simulink model "Final_Simulink_Model_assignment_2"  (R2022b)
settings: Solver=FixedStepAuto  StartTime=0.0  StopTime=inf  FixedStep=1e-3  RelTol=1e-3  EnableMultiTasking=on
undefined symbols (not defined in the file): ATR_PULSE_WIDTH, ATR_PUSLE_WIDTH, D0, D1, D10, D11, D12, D13, D2, D3, D4, D5, D6, D7, D8, D9, LRL, magnitude, PTA0, PTA1, PTA2, PTB23, PTB9, PTC16, PTC17, PTC2, PTC3, PTC4, PTD0, PTD1, PTD2, PTD3, REF_PERIOD, REF_PREIOD, VENT_PULSE_WIDTH
libraries: frdmk64flib x19, etargetslib x9, dspstat3 x1
settings Model: ExtModeTrigDuration=5  Creator=clara  LastModifiedBy=dinghao
settings OptimizationCC: EnhancedBackFolding=on  PassReuseOutputArgsAs=Individual arguments  ZeroExternalMemoryAtStartup=off  ZeroInternalMemoryAtStartup=off  MaxStackSize=64  OptimizeBlockOrder=speed  DifferentSizesBufferReuse=on  OptimizationCustomize=off  EfficientTunableParamExpr=on
settings DebuggingCC: ParameterTunabilityLossMsg=error
settings HardwareCC: ProdBitPerPointer=32  ProdBitPerSizeT=32  ProdBitPerPtrDiffT=32  ProdLargestAtomicInteger=Long  ProdLargestAtomicFloat=Double  ProdWordSize=32  ProdHWDeviceType=ARM Compatible->ARM Cortex
settings ModelReferenceCC: EnableRefExpFcnMdlSchedulingChecks=on
settings SFSimCC: MATLABDynamicMemAlloc=off
settings RTWCC: Description=Embedded Coder  SystemTargetFile=ert.tlc  HardwareBoard=NXP FRDM-K64F  TLCOptions="-aInlineSetEventsForThisBaseRateFcn=TLC_FALSE -aSuppressMultiTaskScheduler=TLC_FALSE  -aRateBasedStepFcn=0"  TemplateMakefile=ert_default_tmf  Toolchain=GNU Tools for ARM Embedded Processors
settings CodeAppCC: ForceParamTrailComments=on  IgnoreCustomStorageClasses=off  OperatorAnnotations=on  SimulinkDataObjDesc=on  SFDataObjDesc=on  InsertBlockDesc=on
settings ERTTargetCC: ExtModeTransport=4  ExtModeMexFile=sendToCommService

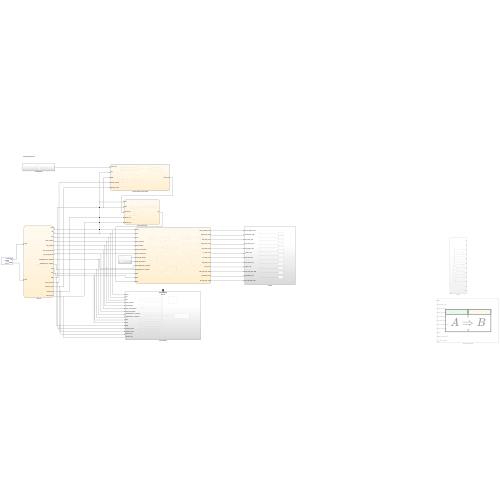
[thumbnail: Simulink's stored preview of the top-level diagram]
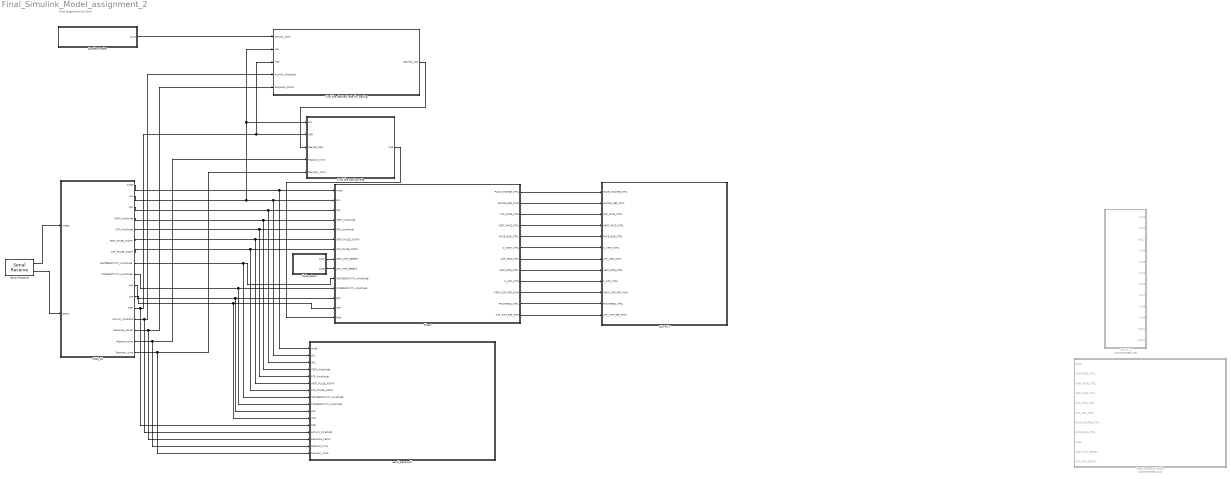
== system Final_Simulink_Model_assignment_2 ==
  note: Find target activity level
  Accelerometer : Subsystem
  COM_IN : Stateflow chart  TreatAsAtomicUnit=on
  Chart : Stateflow chart  TreatAsAtomicUnit=on
      settings: PortSchema="{\"entries\":[{\"content\":{\"sides\":[{\"content\":{\"connectorIds\":[\"In10\",\"In1\",\"In6\",\"In2\",\"In3\",\"In4\",\"In5\",\"In7\",\"In8\",\"In9\",\"In11\",\"In12\",\"In13\",\"In14\"]},\"type\":\"ConnectorPlacement.EquallySpacedRectSide\",\"uuid\":\"411cfc43-89c3-4653-9fab-0da98be593d3\"},{\"content\":{\"connectorIds\":[\"Out1\",\"Out2\",\"Out3\",\"Out4\",\"Out5\",\"Out6\",\"Out7\",\"Out8\",\"Out9\",\"Out10\",\"Out11\",\"Out12\"],\"side\":\"RIGHT\"},\"type\":\"ConnectorPlacement.EquallySpacedRectSide\",\"uuid\":\"ad1683f7-26aa-4767-b656-f3b731cb8235\"},{\"content\":{\"connectorIds\":[],\"side\":\"TOP\"},\"type\":\"ConnectorPlacement.EquallySpacedRectSide\",\"uuid\":\"fbccba07-c1cc-4c9f-8e56-0bdfb6912bb8\"}]},\"type\":\"ConnectorPlacement.EquallySpacedConnector\",\"uuid\":\"0c618a7f-9484-4de3-a6ac-3c8308721375\"}],\"packageUris\":[\"http://schema.mathworks.com/mf0/Connector/R2020b\"],\"version\":\"1.0\"}"
  Find the desired rate for pacing : Stateflow chart  TreatAsAtomicUnit=on
  Find the pacing rate : Stateflow chart  TreatAsAtomicUnit=on
  INPUT 1 : Subsystem  Commented=on
  OUTPUT : Subsystem
  Requirements Table : Requirements Table  Commented=on  TreatAsAtomicUnit=on
  Serial Receive : frdmk64flib/Serial Receive  SCIModule=0  Baudrate=uint32(9600)  Parity=None  StopBits=1  HardwareFlowControl=None  ByteOrder=LittleEndian  DataType=uint8  DataLength=49  BlockingMode=off  OutputStatus=on  SampleTime=-1
  Subsystem : Subsystem
  send_params() : Subsystem
  wires:
  Chart/7(ATR_GND_CTRL) -> OUTPUT/7(ATR_GND_CTRL)
  Chart/3(ATR_PACE_CTRL) -> OUTPUT/3(ATR_PACE_CTRL)
  Chart/6(Z_VENT_CTRL) -> OUTPUT/6(Z_VENT_CTRL)
  Chart/8(VENT_GND_CTRL) -> OUTPUT/8(VENT_GND_CTRL)
  Chart/5(PACE_GND_CTRL) -> OUTPUT/5(PACE_GND_CTRL)
  Chart/9(Z_ATR_CTRL) -> OUTPUT/9(Z_ATR_CTRL)
  Chart/2(PACING_REF_PWM) -> OUTPUT/2(PACING_REF_PWM)
  Chart/1(PACE_CHARGE_CTRL) -> OUTPUT/1(PACE_CHARGE_CTRL)
  Chart/4(VENT_PACE_CTRL) -> OUTPUT/4(VENT_PACE_CTRL)
  Chart/11(FRONTEND_CTRL) -> OUTPUT/11(FRONTEND_CTRL)
  Chart/10(VENT_CMP_REF_PWM) -> OUTPUT/10(VENT_CMP_REF_PWM)
  Chart/12(ATR_CMP_REF_PWM) -> OUTPUT/12(ATR_CMP_REF_PWM)
  Serial Receive/1 -> COM_IN/1(rxdata)
  Serial Receive/2 -> COM_IN/2(status)
  Accelerometer/1(Out1) -> Find the desired rate for pacing/1(Activity_level)
  COM_IN/2(LRL) -> send_params()/2(LRL), Chart/1(LRL), Find the pacing rate/1(LRL), Find the desired rate for pacing/2(LRL)
  COM_IN/12(MSR) -> send_params()/12(MSR), Find the pacing rate/2(MSR), Find the desired rate for pacing/3(MSR)
  COM_IN/13(Activity_threshold) -> send_params()/13(Activity_threshold), Find the desired rate for pacing/4(Activity_threshold)
  COM_IN/14(Response_Factor) -> send_params()/14(Response_Factor), Find the desired rate for pacing/5(Response_Factor)
  Find the desired rate for pacing/1(Desired_rate) -> Find the pacing rate/3(Desired_rate)
  COM_IN/15(Reaction_time) -> send_params()/15(Reaction_time), Find the pacing rate/4(Reaction_time)
  COM_IN/16(Recovery_time) -> send_params()/16(Recovery_time), Find the pacing rate/5(Recovery_time)
  Find the pacing rate/1(rate) -> Chart/14(Rate)
  COM_IN/1(mode) -> send_params()/1(mode), Chart/10(mode)
  COM_IN/3(URL) -> send_params()/3(URL), Chart/6(URL)
  COM_IN/4(VENT_Amplitude) -> send_params()/4(VENT_Amplitude), Chart/2(VENT_Amplitude)
  COM_IN/5(ATR_Amplitude) -> send_params()/5(ATR_Amplitude), Chart/3(ATR_Amplitude)
  COM_IN/6(VENT_PULSE_WIDTH) -> send_params()/6(VENT_PULSE_WIDTH), Chart/4(VENT_PULSE_WIDTH)
  COM_IN/7(ATR_PULSE_WIDTH) -> send_params()/7(ATR_PULSE_WIDTH), Chart/5(ATR_PULSE_WIDTH)
  COM_IN/8(VENTSENSITIVITY_Amplitude) -> send_params()/8(VENTSENSITIVITY_Amplitude), Chart/9(VENTSENSITIVITY_Amplitude)
  COM_IN/9(ATRSENSITIVITY_Amplitude) -> send_params()/9(ATRSENSITIVITY_Amplitude), Chart/11(ATRSENSITIVITY_Amplitude)
  Subsystem/1(Out7) -> Chart/7(VENT_CMP_DETECT)
  Subsystem/2(Out8) -> Chart/8(ATR_CMP_DETECT)
  COM_IN/10(ARP) -> send_params()/10(ARP), Chart/12(ARP)
  COM_IN/11(VRP) -> send_params()/11(VRP), Chart/13(VRP)

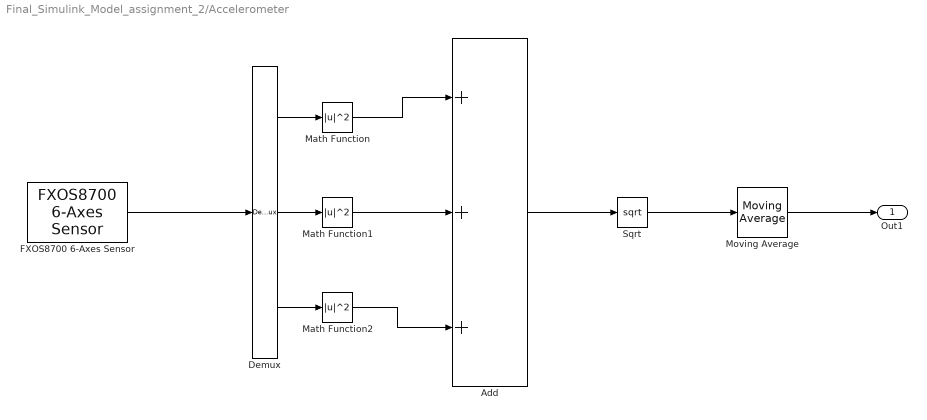
== system Final_Simulink_Model_assignment_2/Accelerometer ==
  Add : Sum  Inputs=+++
  Demux : Demux  Outputs=3
  FXOS8700 6-Axes Sensor : frdmk64flib/FXOS8700 6-Axes Sensor  Activesensor=Accelerometer only  ODR=800Hz  HybridODR=400Hz  Accelfullrange=-4g to +4g  SampleTime=0.01
  Math Function : Math  Operator=magnitude^2
  Math Function1 : Math  Operator=magnitude^2
  Math Function2 : Math  Operator=magnitude^2
  Moving Average : dspstat3/Moving Average  Method=Sliding window  ForgettingFactorPort=off  SpecifyWindowLength=on  WindowLength=4  OverlapLength=3  AllowArbitraryInputLength=off  ForgettingFactor=0.9  SimulateUsing=Code generation
  Sqrt : Sqrt
  Out1 : Outport
  wires:
  FXOS8700 6-Axes Sensor/1 -> Demux/1
  Demux/1 -> Math Function/1
  Demux/2 -> Math Function1/1
  Demux/3 -> Math Function2/1
  Math Function/1 -> Add/1
  Math Function2/1 -> Add/3
  Math Function1/1 -> Add/2
  Add/1 -> Sqrt/1
  Sqrt/1 -> Moving Average/1
  Moving Average/1 -> Out1/1

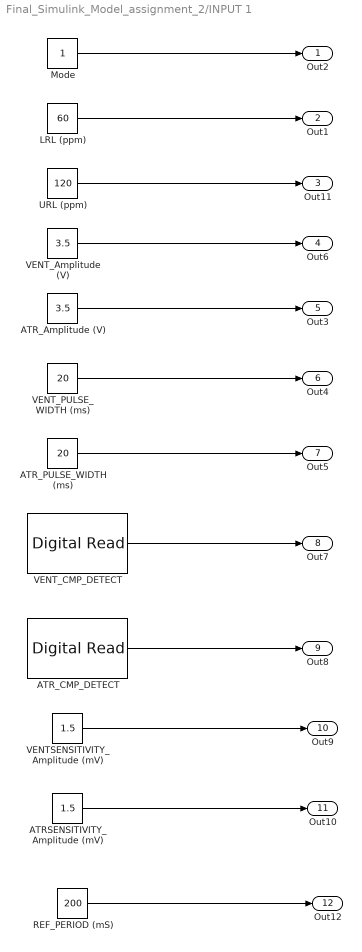
== system Final_Simulink_Model_assignment_2/INPUT 1 ==
  ATRSENSITIVITY_Amplitude (mV) : Constant  Value=1.5
  ATR_Amplitude (V) : Constant  Value=3.5
  ATR_CMP_DETECT : frdmk64flib/Digital Read  Whichpin=PTC16 (D0)  SampleTime=-1
  ATR_PULSE_WIDTH (ms) : Constant  Value=20
  LRL (ppm) : Constant  Value=60
  Mode : Constant
  REF_PERIOD (mS) : Constant  Value=200
  URL (ppm) : Constant  Value=120
  VENTSENSITIVITY_Amplitude (mV) : Constant  Value=1.5
  VENT_Amplitude (V) : Constant  Value=3.5
  VENT_CMP_DETECT : frdmk64flib/Digital Read  Whichpin=PTC17 (D1)  SampleTime=-1
  VENT_PULSE_WIDTH (ms) : Constant  Value=20
  Out2 : Outport
  Out1 : Outport  Port=2
  Out11 : Outport  Port=3
  Out6 : Outport  Port=4
  Out3 : Outport  Port=5
  Out4 : Outport  Port=6
  Out5 : Outport  Port=7
  Out7 : Outport  Port=8
  Out8 : Outport  Port=9
  Out9 : Outport  Port=10
  Out10 : Outport  Port=11
  Out12 : Outport  Port=12
  wires:
  LRL (ppm)/1 -> Out1/1
  VENT_PULSE_WIDTH (ms)/1 -> Out4/1
  VENT_Amplitude (V)/1 -> Out6/1
  URL (ppm)/1 -> Out11/1
  Mode/1 -> Out2/1
  ATR_Amplitude (V)/1 -> Out3/1
  ATR_PULSE_WIDTH (ms)/1 -> Out5/1
  VENT_CMP_DETECT/1 -> Out7/1
  ATR_CMP_DETECT/1 -> Out8/1
  VENTSENSITIVITY_Amplitude (mV)/1 -> Out9/1
  ATRSENSITIVITY_Amplitude (mV)/1 -> Out10/1
  REF_PERIOD (mS)/1 -> Out12/1

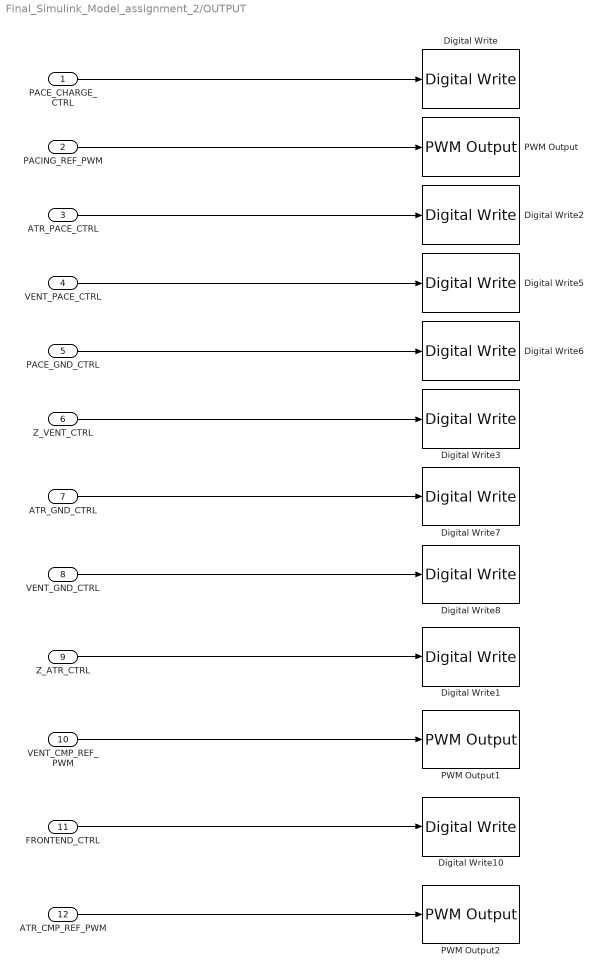
== system Final_Simulink_Model_assignment_2/OUTPUT ==
  PACE_CHARGE_CTRL : Inport
  PACING_REF_PWM : Inport  Port=2
  ATR_PACE_CTRL : Inport  Port=3
  VENT_PACE_CTRL : Inport  Port=4
  PACE_GND_CTRL : Inport  Port=5
  Z_VENT_CTRL : Inport  Port=6
  ATR_GND_CTRL : Inport  Port=7
  VENT_GND_CTRL : Inport  Port=8
  Z_ATR_CTRL : Inport  Port=9
  VENT_CMP_REF_PWM : Inport  Port=10
  FRONTEND_CTRL : Inport  Port=11
  ATR_CMP_REF_PWM : Inport  Port=12
  Digital Write : frdmk64flib/Digital Write  Whichpin=PTB9 (D2)
  Digital Write1 : frdmk64flib/Digital Write  Whichpin=PTB23 (D4)
  Digital Write10 : frdmk64flib/Digital Write  Whichpin=PTD1 (D13)
  Digital Write2 : frdmk64flib/Digital Write  Whichpin=PTA0 (D8)
  Digital Write3 : frdmk64flib/Digital Write  Whichpin=PTC3 (D7)
  Digital Write5 : frdmk64flib/Digital Write  Whichpin=PTC4 (D9)
  Digital Write6 : frdmk64flib/Digital Write  Whichpin=PTD0 (D10)
  Digital Write7 : frdmk64flib/Digital Write  Whichpin=PTD2 (D11)
  Digital Write8 : frdmk64flib/Digital Write  Whichpin=PTD3 (D12)
  PWM Output : frdmk64flib/PWM Output  Whichpin=PTA2 (D5)  InitialFrequency=2000  InitialDutyCycle=0
  PWM Output1 : frdmk64flib/PWM Output  Whichpin=PTA1 (D3)  InitialFrequency=2000  InitialDutyCycle=0
  PWM Output2 : frdmk64flib/PWM Output  Whichpin=PTC2 (D6)  InitialFrequency=2000  InitialDutyCycle=0
  wires:
  PACE_CHARGE_CTRL/1 -> Digital Write/1
  PACING_REF_PWM/1 -> PWM Output/1
  ATR_PACE_CTRL/1 -> Digital Write2/1
  VENT_PACE_CTRL/1 -> Digital Write5/1
  PACE_GND_CTRL/1 -> Digital Write6/1
  Z_VENT_CTRL/1 -> Digital Write3/1
  ATR_GND_CTRL/1 -> Digital Write7/1
  VENT_GND_CTRL/1 -> Digital Write8/1
  Z_ATR_CTRL/1 -> Digital Write1/1
  VENT_CMP_REF_PWM/1 -> PWM Output1/1
  FRONTEND_CTRL/1 -> Digital Write10/1
  ATR_CMP_REF_PWM/1 -> PWM Output2/1

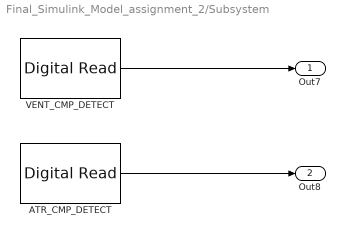
== system Final_Simulink_Model_assignment_2/Subsystem ==
  ATR_CMP_DETECT : frdmk64flib/Digital Read  Whichpin=PTC16 (D0)  SampleTime=-1
  VENT_CMP_DETECT : frdmk64flib/Digital Read  Whichpin=PTC17 (D1)  SampleTime=-1
  Out7 : Outport
  Out8 : Outport  Port=2
  wires:
  ATR_CMP_DETECT/1 -> Out8/1
  VENT_CMP_DETECT/1 -> Out7/1

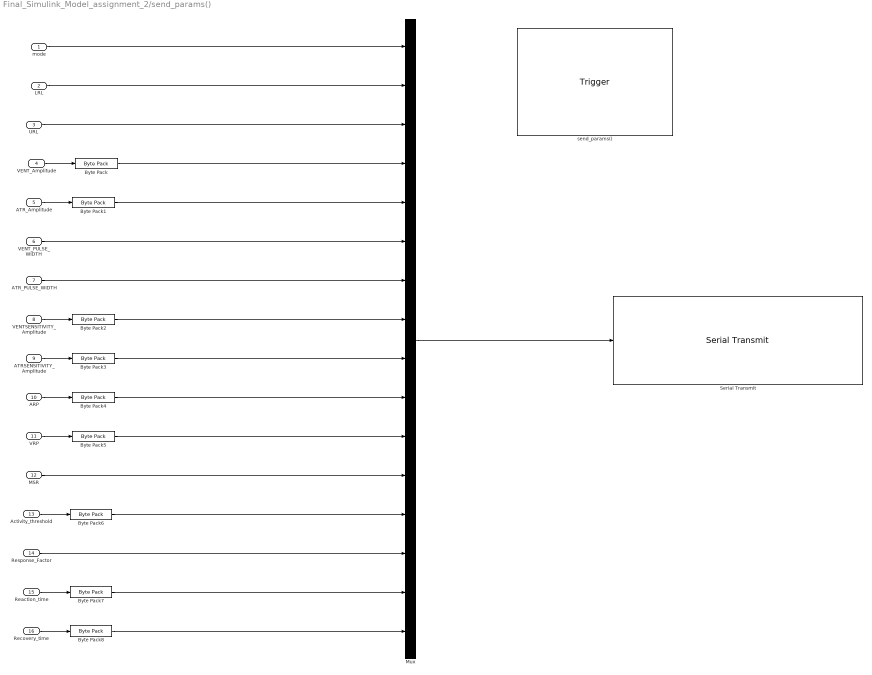
== system Final_Simulink_Model_assignment_2/send_params() ==
  mode : Inport
  LRL : Inport  Port=2
  URL : Inport  Port=3
  VENT_Amplitude : Inport  Port=4
  ATR_Amplitude : Inport  Port=5
  VENT_PULSE_WIDTH : Inport  Port=6
  ATR_PULSE_WIDTH : Inport  Port=7
  VENTSENSITIVITY_Amplitude : Inport  Port=8
  ATRSENSITIVITY_Amplitude : Inport  Port=9
  ARP : Inport  Port=10
  VRP : Inport  Port=11
  MSR : Inport  Port=12
  Activity_threshold : Inport  Port=13
  Response_Factor : Inport  Port=14
  Reaction_time : Inport  Port=15
  Recovery_time : Inport  Port=16
  send_params() : TriggerPort  TriggerType=function-call  IsSimulinkFunction=on  FunctionName=send_params  VariantControl=Variant
  Byte Pack{,1..3,6} (5 alike) : etargetslib/Byte Pack  datatypes={'single'}  byteAlign=1
  Byte Pack4 : etargetslib/Byte Pack  datatypes={'uint16'}  byteAlign=1
  Byte Pack5 : etargetslib/Byte Pack  datatypes={'uint16'}  byteAlign=1
  Byte Pack7 : etargetslib/Byte Pack  datatypes={'double'}  byteAlign=1
  Byte Pack8 : etargetslib/Byte Pack  datatypes={'double'}  byteAlign=1
  Mux : Mux  Inputs=16
  Serial Transmit : frdmk64flib/Serial Transmit  SCIModule=0  Baudrate=uint32(9600)  Parity=None  StopBits=1  HardwareFlowControl=None  ByteOrder=LittleEndian  BlockingMode=on  OutputStatus=off
  wires:
  mode/1 -> Mux/1
  LRL/1 -> Mux/2
  URL/1 -> Mux/3
  VENT_Amplitude/1 -> Byte Pack/1
  Byte Pack/1 -> Mux/4
  ATR_Amplitude/1 -> Byte Pack1/1
  Byte Pack1/1 -> Mux/5
  VENT_PULSE_WIDTH/1 -> Mux/6
  ATR_PULSE_WIDTH/1 -> Mux/7
  VENTSENSITIVITY_Amplitude/1 -> Byte Pack2/1
  Byte Pack2/1 -> Mux/8
  ATRSENSITIVITY_Amplitude/1 -> Byte Pack3/1
  Byte Pack3/1 -> Mux/9
  Byte Pack4/1 -> Mux/10
  ARP/1 -> Byte Pack4/1
  VRP/1 -> Byte Pack5/1
  Byte Pack5/1 -> Mux/11
  MSR/1 -> Mux/12
  Activity_threshold/1 -> Byte Pack6/1
  Byte Pack6/1 -> Mux/13
  Response_Factor/1 -> Mux/14
  Byte Pack7/1 -> Mux/15
  Reaction_time/1 -> Byte Pack7/1
  Byte Pack8/1 -> Mux/16
  Recovery_time/1 -> Byte Pack8/1
  Mux/1 -> Serial Transmit/1

== stateflow chart Final_Simulink_Model_assignment_2/Requirements Table ==
  (default) -> (junction 1073743363)
  (junction 1073743363) -> (junction 1073743364) : {
      | % SF_REQ_REV_07
      | }
  (junction 1073743364) -> (junction 1073743366) : {
      | % HEADER_ASSIGNMENTS
      |
      | }
  (junction 1073743366) -> (junction 1073743368) : {
      | % START_A_4
      | }
  (junction 1073743368) -> (junction 1073743370) : {
      | }
  (junction 1073743370) -> (junction 1073743372)
  (junction 1073743372) -> (junction 1073743374) : {
      | }
  (junction 1073743374) -> (junction 1073743376) : {
      | % END_A_4
      | }
  (junction 1073743376) -> (junction 1073743378) : {
      | % START_R_1
      | }
  (junction 1073743378) -> (junction 1073743380) : {
      | }
  (junction 1073743380) -> (junction 1073743382)
  (junction 1073743382) -> (junction 1073743384) [order 1] : [(((Mode) == (1)))]
  (junction 1073743382) -> (junction 1073743426) [order 2]
  (junction 1073743384) -> (junction 1073743386) : {
      |
      |
      | }
  (junction 1073743386) -> (junction 1073743388) : {
      | }
  (junction 1073743388) -> (junction 1073743390) : {
      | % START_R_7
      | }
  (junction 1073743390) -> (junction 1073743392) : {
      | }
  (junction 1073743392) -> (junction 1073743394)
  (junction 1073743394) -> (junction 1073743396) [order 1] : [duration((((State) == (1)))) >= 60000/LRL - ATR_PUSLE_WIDTH]
  (junction 1073743394) -> (junction 1073743402) [order 2]
  (junction 1073743396) -> (junction 1073743398) : {
      | reqtable_postcondition((((ATR_PACE_CTRL) == (1))) && (((ATR_GND_CTRL) == (0))) && (((PACE_CHARGE_CTRL) == (0))) && (((PACE_GND_CTRL) == (1))), 'R:1.1');
      |
      |
      | }
  (junction 1073743398) -> (junction 1073743400) : {
      | }
  (junction 1073743400) -> (junction 1073743402)
  (junction 1073743402) -> (junction 1073743404)
  (junction 1073743404) -> (junction 1073743406) : {
      | % END_R_7
      | }
  (junction 1073743406) -> (junction 1073743408) : {
      | % START_R_10
      | }
  (junction 1073743408) -> (junction 1073743410) : {
      | }
  (junction 1073743410) -> (junction 1073743412)
  (junction 1073743412) -> (junction 1073743414) [order 1] : [duration((((State) == (2)))) >= ATR_PULSE_WIDTH]
  (junction 1073743412) -> (junction 1073743420) [order 2]
  (junction 1073743414) -> (junction 1073743416) : {
      | reqtable_postcondition((((ATR_PACE_CTRL) == (0))) && (((ATR_GND_CTRL) == (1))) && (((PACE_CHARGE_CTRL) == (1))) && (((PACE_GND_CTRL) == (1))), 'R:1.2');
      |
      |
      | }
  (junction 1073743416) -> (junction 1073743418) : {
      | }
  (junction 1073743418) -> (junction 1073743420)
  (junction 1073743420) -> (junction 1073743422)
  (junction 1073743422) -> (junction 1073743424) : {
      | % END_R_10
      | }
  (junction 1073743424) -> (junction 1073743426)
  (junction 1073743426) -> (junction 1073743428)
  (junction 1073743428) -> (junction 1073743430) : {
      | % END_R_1
      | }
  (junction 1073743430) -> (junction 1073743432) : {
      | % START_R_13
      | }
  (junction 1073743432) -> (junction 1073743434) : {
      | }
  (junction 1073743434) -> (junction 1073743436)
  (junction 1073743436) -> (junction 1073743438) [order 1] : [(((Mode) == (2)))]
  (junction 1073743436) -> (junction 1073743480) [order 2]
  (junction 1073743438) -> (junction 1073743440) : {
      |
      |
      | }
  (junction 1073743440) -> (junction 1073743442) : {
      | }
  (junction 1073743442) -> (junction 1073743444) : {
      | % START_R_16
      | }
  (junction 1073743444) -> (junction 1073743446) : {
      | }
  (junction 1073743446) -> (junction 1073743448)
  (junction 1073743448) -> (junction 1073743450) [order 1] : [duration((((State) == (1)))) >= 60000/LRL - VENT_PULSE_WIDTH]
  (junction 1073743448) -> (junction 1073743456) [order 2]
  (junction 1073743450) -> (junction 1073743452) : {
      | reqtable_postcondition((((PACE_CHARGE_CTRL) == (0))) && (((PACE_GND_CTRL) == (1))) && (((VENT_PACE_CTRL) == (1))) && (((VENT_GND_CTRL) == (0))), 'R:2.1');
      |
      |
      | }
  (junction 1073743452) -> (junction 1073743454) : {
      | }
  (junction 1073743454) -> (junction 1073743456)
  (junction 1073743456) -> (junction 1073743458)
  (junction 1073743458) -> (junction 1073743460) : {
      | % END_R_16
      | }
  (junction 1073743460) -> (junction 1073743462) : {
      | % START_R_19
      | }
  (junction 1073743462) -> (junction 1073743464) : {
      | }
  (junction 1073743464) -> (junction 1073743466)
  (junction 1073743466) -> (junction 1073743468) [order 1] : [duration((((State) == (2)))) >= VENT_PULSE_WIDTH]
  (junction 1073743466) -> (junction 1073743474) [order 2]
  (junction 1073743468) -> (junction 1073743470) : {
      | reqtable_postcondition((((PACE_CHARGE_CTRL) == (1))) && (((PACE_GND_CTRL) == (1))) && (((VENT_PACE_CTRL) == (0))) && (((VENT_GND_CTRL) == (1))), 'R:2.2');
      |
      |
      | }
  (junction 1073743470) -> (junction 1073743472) : {
      | }
  (junction 1073743472) -> (junction 1073743474)
  (junction 1073743474) -> (junction 1073743476)
  (junction 1073743476) -> (junction 1073743478) : {
      | % END_R_19
      | }
  (junction 1073743478) -> (junction 1073743480)
  (junction 1073743480) -> (junction 1073743482)
  (junction 1073743482) -> (junction 1073743484) : {
      | % END_R_13
      | }
  (junction 1073743484) -> (junction 1073743486) : {
      | % START_R_22
      | }
  (junction 1073743486) -> (junction 1073743488) : {
      | }
  (junction 1073743488) -> (junction 1073743490)
  (junction 1073743490) -> (junction 1073743492) [order 1] : [(((Mode) == (3)))]
  (junction 1073743490) -> (junction 1073743552) [order 2]
  (junction 1073743492) -> (junction 1073743494) : {
      |
      |
      | }
  (junction 1073743494) -> (junction 1073743496) : {
      | }
  (junction 1073743496) -> (junction 1073743498) : {
      | % START_R_25
      | }
  (junction 1073743498) -> (junction 1073743500) : {
      | }
  (junction 1073743500) -> (junction 1073743502)
  (junction 1073743502) -> (junction 1073743504) [order 1] : [duration((((State) == (1)))) >= 60000/LRL - ATR_PULSE_WIDTH]
  (junction 1073743502) -> (junction 1073743510) [order 2]
  (junction 1073743504) -> (junction 1073743506) : {
      | reqtable_postcondition((((ATR_PACE_CTRL) == (0))) && (((ATR_GND_CTRL) == (1))) && (((PACE_CHARGE_CTRL) == (1))) && (((PACE_GND_CTRL) == (1))) && (((FRONTEND_CTRL) == (1))), 'R:3.1');
      |
      |
      | }
  (junction 1073743506) -> (junction 1073743508) : {
      | }
  (junction 1073743508) -> (junction 1073743510)
  (junction 1073743510) -> (junction 1073743512)
  (junction 1073743512) -> (junction 1073743514) : {
      | % END_R_25
      | }
  (junction 1073743514) -> (junction 1073743516) : {
      | % START_R_28
      | }
  (junction 1073743516) -> (junction 1073743518) : {
      | }
  (junction 1073743518) -> (junction 1073743520)
  (junction 1073743520) -> (junction 1073743522) [order 1] : [duration((((State) == (2)))) >= ATR_PULSE_WIDTH]
  (junction 1073743520) -> (junction 1073743528) [order 2]
  (junction 1073743522) -> (junction 1073743524) : {
      | reqtable_postcondition((((ATR_PACE_CTRL) == (1))) && (((ATR_GND_CTRL) == (0))) && (((PACE_CHARGE_CTRL) == (0))) && (((PACE_GND_CTRL) == (1))), 'R:3.2');
      |
      |
      | }
  (junction 1073743524) -> (junction 1073743526) : {
      | }
  (junction 1073743526) -> (junction 1073743528)
  (junction 1073743528) -> (junction 1073743530)
  (junction 1073743530) -> (junction 1073743532) : {
      | % END_R_28
      | }
  (junction 1073743532) -> (junction 1073743534) : {
      | % START_R_31
      | }
  (junction 1073743534) -> (junction 1073743536) : {
      | }
  (junction 1073743536) -> (junction 1073743538)
  (junction 1073743538) -> (junction 1073743540) [order 1] : [duration((((State) == (3)))) >= REF_PERIOD]
  (junction 1073743538) -> (junction 1073743546) [order 2]
  (junction 1073743540) -> (junction 1073743542) : {
      | reqtable_postcondition((((ATR_PACE_CTRL) == (0))) && (((ATR_GND_CTRL) == (1))) && (((PACE_CHARGE_CTRL) == (0))) && (((PACE_GND_CTRL) == (1))) && (((FRONTEND_CTRL) == (0))), 'R:3.3');
      |
      |
      | }
  (junction 1073743542) -> (junction 1073743544) : {
      | }
  (junction 1073743544) -> (junction 1073743546)
  (junction 1073743546) -> (junction 1073743548)
  (junction 1073743548) -> (junction 1073743550) : {
      | % END_R_31
      | }
  (junction 1073743550) -> (junction 1073743552)
  (junction 1073743552) -> (junction 1073743554)
  (junction 1073743554) -> (junction 1073743556) : {
      | % END_R_22
      | }
  (junction 1073743556) -> (junction 1073743558) : {
      | % START_R_34
      | }
  (junction 1073743558) -> (junction 1073743560) : {
      | }
  (junction 1073743560) -> (junction 1073743562)
  (junction 1073743562) -> (junction 1073743564) [order 1] : [(((Mode) == (4)))]
  (junction 1073743562) -> (junction 1073743624) [order 2]
  (junction 1073743564) -> (junction 1073743566) : {
      |
      |
      | }
  (junction 1073743566) -> (junction 1073743568) : {
      | }
  (junction 1073743568) -> (junction 1073743570) : {
      | % START_R_37
      | }
  (junction 1073743570) -> (junction 1073743572) : {
      | }
  (junction 1073743572) -> (junction 1073743574)
  (junction 1073743574) -> (junction 1073743576) [order 1] : [duration((((State) == (1)))) >= 60000/LRL - VENT_PULSE_WIDTH]
  (junction 1073743574) -> (junction 1073743582) [order 2]
  (junction 1073743576) -> (junction 1073743578) : {
      | reqtable_postcondition((((PACE_CHARGE_CTRL) == (1))) && (((PACE_GND_CTRL) == (1))) && (((VENT_PACE_CTRL) == (0))) && (((VENT_GND_CTRL) == (1))) && (((FRONTEND_CTRL) == (1))), 'R:4.1');
      |
      |
      | }
  (junction 1073743578) -> (junction 1073743580) : {
      | }
  (junction 1073743580) -> (junction 1073743582)
  (junction 1073743582) -> (junction 1073743584)
  (junction 1073743584) -> (junction 1073743586) : {
      | % END_R_37
      | }
  (junction 1073743586) -> (junction 1073743588) : {
      | % START_R_40
      | }
  (junction 1073743588) -> (junction 1073743590) : {
      | }
  (junction 1073743590) -> (junction 1073743592)
  (junction 1073743592) -> (junction 1073743594) [order 1] : [duration((((State) == (2)))) >= VENT_PULSE_WIDTH]
  (junction 1073743592) -> (junction 1073743600) [order 2]
  (junction 1073743594) -> (junction 1073743596) : {
      | reqtable_postcondition((((PACE_CHARGE_CTRL) == (0))) && (((PACE_GND_CTRL) == (1))) && (((VENT_PACE_CTRL) == (1))) && (((VENT_GND_CTRL) == (0))), 'R:4.2');
      |
      |
      | }
  (junction 1073743596) -> (junction 1073743598) : {
      | }
  (junction 1073743598) -> (junction 1073743600)
  (junction 1073743600) -> (junction 1073743602)
  (junction 1073743602) -> (junction 1073743604) : {
      | % END_R_40
      | }
  (junction 1073743604) -> (junction 1073743606) : {
      | % START_R_43
      | }
  (junction 1073743606) -> (junction 1073743608) : {
      | }
  (junction 1073743608) -> (junction 1073743610)
  (junction 1073743610) -> (junction 1073743612) [order 1] : [duration((((State) == (3)))) >= REF_PREIOD]
  (junction 1073743610) -> (junction 1073743618) [order 2]
  (junction 1073743612) -> (junction 1073743614) : {
      | reqtable_postcondition((((PACE_CHARGE_CTRL) == (0))) && (((PACE_GND_CTRL) == (1))) && (((VENT_PACE_CTRL) == (0))) && (((VENT_GND_CTRL) == (1))) && (((FRONTEND_CTRL) == (0))), 'R:4.3');
      |
      |
      | }
  (junction 1073743614) -> (junction 1073743616) : {
      | }
  (junction 1073743616) -> (junction 1073743618)
  (junction 1073743618) -> (junction 1073743620)
  (junction 1073743620) -> (junction 1073743622) : {
      | % END_R_43
      | }
  (junction 1073743622) -> (junction 1073743624)
  (junction 1073743624) -> (junction 1073743626)
  (junction 1073743626) -> (junction 1073743628) : {
      | % END_R_34
      | }
  data: State input; FRONTEND_CTRL input; VENT_PACE_CTRL input; VENT_GND_CTRL input; ATR_PACE_CTRL input; ATR_GND_CTRL input; PACE_CHARGE_CTRL input; PACE_GND_CTRL input; Mode input double; VENT_CMP_DETECT input; ATR_CMP_DETECT input; ATR_PULSE_WIDTH parameter; LRL parameter; ATR_PUSLE_WIDTH parameter; VENT_PULSE_WIDTH parameter; REF_PREIOD parameter; REF_PERIOD parameter

== stateflow chart Final_Simulink_Model_assignment_2/COM_IN ==
  settings: executeAtInitialization=1
  state SET_PARAM
    entry:
    mode = rxdata(3);
    LRL = rxdata(4);
    URL = rxdata(5);
    VENT_Amplitude = typecast(rxdata(6:9),'single');
    ATR_Amplitude = typecast(rxdata(10:13),'single');
    VENT_PULSE_WIDTH = rxdata(14);
    ATR_PULSE_WIDTH = rxdata(15);
    VENTSENSITIVITY_Amplitude = typecast(rxdata(16:19),'single');
    ATRSENSITIVITY_Amplitude = typecast(rxdata(20:23),'single');
    ARP = typecast(rxdata(24:25),'uint16');
    VRP = typecast(rxdata(26:27),'uint16');
    MSR = rxdata(28);
    Activity_threshold = typecast(rxdata(29:32),'single');
    Response_Factor = rxdata(33);
    Reaction_time = typecast(rxdata(34:41),'double');
    Recovery_time = typecast(rxdata(42:49),'double');
  state Initialize
    entry:
    mode = 1; % 8 modes in total [1,8]
    LRL = 60; %ppm
    URL = 120; %ppm
    VENT_Amplitude = 3.5; %V
    ATR_Amplitude = 3.5; %V
    VENT_PULSE_WIDTH = 10; % ms
    ATR_PULSE_WIDTH = 10; % ms
    VENTSENSITIVITY_Amplitude = 1.5; %mV
    ATRSENSITIVITY_Amplitude = 1.5; %mV
    ARP = 250; %ms
    VRP = 250; %ms
    MSR = 120; % ppm maximum sensor rate
    Activity_threshold = 1.1; % output of accelerometer shell exceed this value
    Response_Factor = 8; % [1,16]
    Reaction_time = 30; % sec
    Recovery_time = 300; %sec
  state STANDBY
    %waiting for COM
  state ECHO_PARAM
    entry:
    send_params();
  (junction 15) -> SET_PARAM [order 1] : [rxdata(2) == hex2dec('55')]
  (default) -> Initialize
  STANDBY -> (junction 13) : [status == 0]
  (junction 13) -> (junction 15) [order 1] : [rxdata(1) == hex2dec('16')]
  (junction 13) -> STANDBY [order 2]
  (junction 15) -> ECHO_PARAM [order 2] : [rxdata(2) == hex2dec('22')]
  Initialize -> STANDBY
  ECHO_PARAM -> STANDBY
  data: rxdata input uint8; status input uint8; mode output uint8; LRL output uint8; URL output uint8; VENT_Amplitude output single; ATR_Amplitude output single; VENT_PULSE_WIDTH output uint8; ATR_PULSE_WIDTH output uint8; VENTSENSITIVITY_Amplitude output single; ATRSENSITIVITY_Amplitude output single; ARP output uint16; VRP output uint16; MSR output uint8; Activity_threshold output single; Response_Factor output uint8; Reaction_time output double; Recovery_time output double

== stateflow chart Final_Simulink_Model_assignment_2/Chart ==
  note: Pace ready
  state Pacing_AOO
    entry:
    PACE_CHARGE_CTRL = false;
    PACE_GND_CTRL = true;
    ATR_PACE_CTRL = true;
    ATR_GND_CTRL = false;
    %
  state AOO
    entry:
    % charge condition for C22
    ATR_PACE_CTRL = false;
    PACE_CHARGE_CTRL = true;
    % discharge condition for C21;
    ATR_GND_CTRL = true;
    PACE_GND_CTRL = true;
    %
    PACING_REF_PWM = 20*ATR_Amplitude;
  note: Pace ready
  state AOOR
    entry:
    % charge condition for C22
    ATR_PACE_CTRL = false;
    PACE_CHARGE_CTRL = true;
    % discharge condition for C21;
    ATR_GND_CTRL = true;
    PACE_GND_CTRL = true;
    %
    PACING_REF_PWM = 20*ATR_Amplitude;
  state Pacing_AOOR
    entry:
    PACE_CHARGE_CTRL = false;
    PACE_GND_CTRL = true;
    ATR_PACE_CTRL = true;
    ATR_GND_CTRL = false;
    %
  note: Recharge ready
  note: Recharge ready
  note: Charge C22 and discharge blocking capacitor
  note: Discharge C22 into atrium (charge C21)
  note: Pace ready
  state VOO
    entry:
    % charge condition for C22
    VENT_PACE_CTRL = false;
    PACE_CHARGE_CTRL = true;
    % discharge condition for C21;
    VENT_GND_CTRL = true;
    PACE_GND_CTRL = true;
    %
    PACING_REF_PWM = 20*VENT_Amplitude;
  state Pacing_VOO
    entry:
    PACE_CHARGE_CTRL = false;
    PACE_GND_CTRL = true;
    VENT_GND_CTRL = false;
    VENT_PACE_CTRL = true;
    %
  note: Initial conditions
  state MAIN
    entry:
    VENT_GND_CTRL=false;
    Z_ATR_CTRL = false;
    Z_VENT_CTRL = false;
    FRONTEND_CTRL=false;
    PACE_CHARGE_CTRL = false;
    VENT_PACE_CTRL = false;
    ATR_PACE_CTRL = false;
    PACE_GND_CTRL=false;
    ATR_GND_CTRL=false;
  note: Pace ready
  note: Recharge ready
  state VOOR
    entry:
    % charge condition for C22
    VENT_PACE_CTRL = false;
    PACE_CHARGE_CTRL = true;
    % discharge condition for C21;
    VENT_GND_CTRL = true;
    PACE_GND_CTRL = true;
    %
    PACING_REF_PWM = 20*VENT_Amplitude;
  state Pacing_VOOR
    entry:
    PACE_CHARGE_CTRL = false;
    PACE_GND_CTRL = true;
    VENT_GND_CTRL = false;
    VENT_PACE_CTRL = true;
    %
  note: Charge C22 and discharge blocking capacitor
  note: Discharge C22 into ventrical (charge C21)
  note: Begin sensing, charge C22 and discharge
      | blocking capacitor
  note: Discharge C22 into atrium (charge C21)
  note: If no signal is sensed
  state AAI
    entry:
    % begin sensing
    FRONTEND_CTRL = true;
    % charge condition for C22
    ATR_PACE_CTRL = false;
    PACE_CHARGE_CTRL = true;
    % discharge condition for C21;
    ATR_GND_CTRL = true;
    PACE_GND_CTRL = true;
    %
    PACING_REF_PWM = 70*ATR_Amplitude;
    ATR_CMP_REF_PWM = 70*ATRSENSITIVITY_Amplitude;
  state Pacing_AAI1
    entry:
    PACE_CHARGE_CTRL = false;
    PACE_GND_CTRL = true;
    ATR_PACE_CTRL = true;
    ATR_GND_CTRL = false;
    %
    PACING_REF_PWM = 70*ATR_Amplitude;
  note: If signal is sensed
  state AAI_REFRACTORY
    entry:
    FRONTEND_CTRL = false;
    ATR_PACE_CTRL = false;
    ATR_GND_CTRL = true;
    PACING_REF_PWM = 70*ATR_Amplitude;
    PACE_CHARGE_CTRL = false;
    PACE_GND_CTRL = true;
  note: If no signal is sensed
  state AAIR
    entry:
    % begin sensing
    FRONTEND_CTRL = true;
    % charge condition for C22
    ATR_PACE_CTRL = false;
    PACE_CHARGE_CTRL = true;
    % discharge condition for C21;
    ATR_GND_CTRL = true;
    PACE_GND_CTRL = true;
    %
    PACING_REF_PWM = 70*ATR_Amplitude;
    ATR_CMP_REF_PWM = 70*ATRSENSITIVITY_Amplitude;
  state Pacing_AAIR
    entry:
    PACE_CHARGE_CTRL = false;
    PACE_GND_CTRL = true;
    ATR_PACE_CTRL = true;
    ATR_GND_CTRL = false;
    %
    PACING_REF_PWM = 70*ATR_Amplitude;
  note: If signal is sensed
  note: Follows events during which senses
      | in the atrium are ignored
  note: If signal is sensed
  note: Begin sensing, charge C22 and discharge
      | blocking capacitor
  note: Discharge C22 into ventrical (charge C21)
  note: If no signal is sensed
  state Pacing_VVI
    entry:
    PACE_CHARGE_CTRL = false;
    PACE_GND_CTRL = true;
    VENT_GND_CTRL = false;
    VENT_PACE_CTRL = true;
    %
    PACING_REF_PWM = 70*VENT_Amplitude;
  state VVI
    entry:
    % begin sensing
    FRONTEND_CTRL = true;
    % charge condition for C22
    VENT_PACE_CTRL = false;
    PACE_CHARGE_CTRL = true;
    % discharge condition for C21;
    VENT_GND_CTRL = true;
    PACE_GND_CTRL = true;
    %
    PACING_REF_PWM = 70*VENT_Amplitude;
    VENT_CMP_REF_PWM = 70*VENTSENSITIVITY_Amplitude;
  state AAIR_REFRACTORY
    entry:
    FRONTEND_CTRL = false;
    ATR_PACE_CTRL = false;
    ATR_GND_CTRL = true;
    PACING_REF_PWM = 70*ATR_Amplitude;
    PACE_CHARGE_CTRL = false;
    PACE_GND_CTRL = true;
  note: If signal is sensed
  note: If signal is sensed
  note: Follows events during which senses
      | in the atrium are ignored
  note: If no signal is sensed
  state Pacing_VVIR
    entry:
    PACE_CHARGE_CTRL = false;
    PACE_GND_CTRL = true;
    VENT_GND_CTRL = false;
    VENT_PACE_CTRL = true;
    %
    PACING_REF_PWM = 70*VENT_Amplitude;
  state VVIR
    entry:
    % begin sensing
    FRONTEND_CTRL = true;
    % charge condition for C22
    VENT_PACE_CTRL = false;
    PACE_CHARGE_CTRL = true;
    % discharge condition for C21;
    VENT_GND_CTRL = true;
    PACE_GND_CTRL = true;
    %
    PACING_REF_PWM = 70*VENT_Amplitude;
    VENT_CMP_REF_PWM = 70*VENTSENSITIVITY_Amplitude;
  state VVI_REFRACTORY
    entry:
    FRONTEND_CTRL = false;
    VENT_GND_CTRL = true;
    PACING_REF_PWM = 70*VENT_Amplitude;
    PACE_CHARGE_CTRL = false;
    PACE_GND_CTRL = true;
  note: If signal is sensed
  note: If signal is sensed
  note: Follows events during which senses
      | in the ventrical are ignored
  state VVIR_REFRACTORY
    entry:
    FRONTEND_CTRL = false;
    VENT_GND_CTRL = true;
    PACING_REF_PWM = 70*VENT_Amplitude;
    PACE_CHARGE_CTRL = false;
    PACE_GND_CTRL = true;
  note: If signal is sensed
  AOO -> Pacing_AOO : after((60000/LRL - ATR_PULSE_WIDTH),msec)
  AOOR -> Pacing_AOOR : [after(60000/Rate - ATR_PULSE_WIDTH,msec)]
  MAIN -> AOO [order 4] : [mode == 1]
  Pacing_AOO -> AOO : [after(ATR_PULSE_WIDTH,msec)]
  Pacing_AOOR -> AOOR : [after(ATR_PULSE_WIDTH,msec)]
  MAIN -> AOOR [order 5] : [mode == 5]
  VOO -> Pacing_VOO : [after(60000/LRL - VENT_PULSE_WIDTH,msec)]
  MAIN -> VOO [order 1] : [mode == 2]
  (default) -> MAIN
  Pacing_VOO -> VOO : [after(VENT_PULSE_WIDTH,msec)]
  VOOR -> Pacing_VOOR : [after(60000/Rate - VENT_PULSE_WIDTH,msec)]
  Pacing_VOOR -> VOOR : [after(VENT_PULSE_WIDTH,msec)]
  MAIN -> AAI [order 3] : [mode == 3]
  MAIN -> VOOR [order 6] : [mode == 6]
  MAIN -> AAIR [order 7] : [mode == 7]
  MAIN -> VVIR [order 8] : [mode == 8]
  MAIN -> VVI [order 2] : [mode == 4]
  AAI -> Pacing_AAI1 [order 1] : [(ATR_CMP_DETECT==false) &&after(60000/LRL - ATR_PULSE_WIDTH,msec)]
  Pacing_AAI1 -> AAI [order 1] : [after(ATR_PULSE_WIDTH,msec)]
  AAI -> AAI_REFRACTORY [order 2] : [ATR_CMP_DETECT == true]
  AAI_REFRACTORY -> AAI : [after(ARP,msec)]
  Pacing_AAI1 -> AAI_REFRACTORY [order 2] : [ATR_CMP_DETECT == true]
  AAIR -> Pacing_AAIR [order 1] : [(ATR_CMP_DETECT==false) &&after(60000/Rate - ATR_PULSE_WIDTH,msec)]
  Pacing_AAIR -> AAIR [order 1] : [after(ATR_PULSE_WIDTH,msec)]
  AAIR -> AAIR_REFRACTORY [order 2] : [ATR_CMP_DETECT == true]
  AAIR_REFRACTORY -> AAIR : [after(ARP,msec)]
  Pacing_AAIR -> AAIR_REFRACTORY [order 2] : [ATR_CMP_DETECT == true]
  VVI -> Pacing_VVI [order 1] : [(VENT_CMP_DETECT==false) &&after(60000/LRL - VENT_PULSE_WIDTH,msec)]
  Pacing_VVI -> VVI [order 1] : [after(VENT_PULSE_WIDTH,msec)]
  VVI -> VVI_REFRACTORY [order 2] : [VENT_CMP_DETECT == true]
  Pacing_VVI -> VVI_REFRACTORY [order 2] : [VENT_CMP_DETECT == true]
  VVI_REFRACTORY -> VVI : [after(VRP,msec)]
  VVIR -> Pacing_VVIR [order 1] : [(VENT_CMP_DETECT==false) &&after(60000/Rate - VENT_PULSE_WIDTH,msec)]
  Pacing_VVIR -> VVIR [order 1] : [after(VENT_PULSE_WIDTH,msec)]
  VVIR -> VVIR_REFRACTORY [order 2] : [VENT_CMP_DETECT == true]
  Pacing_VVIR -> VVIR_REFRACTORY [order 2] : [VENT_CMP_DETECT == true]
  VVIR_REFRACTORY -> VVIR : [after(VRP,msec)]
  data: LRL input; VENT_Amplitude input; ATR_Amplitude input; VENT_PULSE_WIDTH input; ATR_PULSE_WIDTH input; URL input; VENT_CMP_DETECT input; ATR_CMP_DETECT input; VENTSENSITIVITY_Amplitude input; PACE_CHARGE_CTRL output; PACING_REF_PWM output; ATR_PACE_CTRL output; VENT_PACE_CTRL output; PACE_GND_CTRL output; Z_VENT_CTRL output; ATR_GND_CTRL output; VENT_GND_CTRL output; Z_ATR_CTRL output; VENT_CMP_REF_PWM output; FRONTEND_CTRL output; mode input; ATR_CMP_REF_PWM output; ATRSENSITIVITY_Amplitude input; ARP input; VRP input; Rate input

== stateflow chart Final_Simulink_Model_assignment_2/Find the desired rate for pacing ==
  state Desired_rate_output_3
    entry:
    Desired_rate = LRL;
  state Check
    % check how the desired rate is going to change depends on activity level
  state Linear_increase
    entry:
    temp_rate = LRL + Response_Factor*Activity_level;
  state Desired_rate_output_2
    entry:
    Desired_rate = MSR;
  state Desired_rate_output_1
    entry:
    Desired_rate = temp_rate;
  (default) -> Check
  Check -> Desired_rate_output_3 [order 2] : [Activity_level <= Activity_threshold]
  Check -> Linear_increase [order 1] : [Activity_level > Activity_threshold]
  Linear_increase -> Desired_rate_output_2 [order 2] : [temp_rate >= MSR]
  Linear_increase -> Desired_rate_output_1 [order 1] : [temp_rate < MSR]
  data: Activity_level input; LRL input; MSR input; Activity_threshold input; Response_Factor input; Desired_rate output; temp_rate local

== stateflow chart Final_Simulink_Model_assignment_2/Find the pacing rate ==
  state Decreasing
    % using linear function to decrease
    entry:
    rate = LRL;
    during:
    rate = rate  - (MSR-LRL)/Recovery_time;
  state Initial_state
  state Increasing
    % using linear function to increase
    entry:
    rate = LRL;
    during:
    rate = rate + (MSR-LRL)/Reaction_time;
  (default) -> Initial_state
  Initial_state -> Decreasing [order 2] : [LRL > Desired_rate]
  Decreasing -> Initial_state : [LRL == Desired_rate]
  Initial_state -> Increasing [order 1] : [LRL < Desired_rate]
  Increasing -> Initial_state : [LRL == Desired_rate]
  data: LRL input; MSR input; Desired_rate input; Reaction_time input; Recovery_time input; rate output
